simulink model "pr743_QPSK_synch_baseband"  (R2018b)
settings: Solver=VariableStepAuto  StartTime=0.0  StopTime=50000/fs  RelTol=1e-3
PreLoadFcn:
  | Rbit   = 100e3;    % битовая скорость
  | Rsyml = Rbit/2;    % символьная скорость
  | fs = 2.4e6;        % частота дискретизации АЦП
  | interp = fs/Rsyml; % коэффициент передискретизации
  | fc = 600e3;        % несущая частота, Гц
  | fe = 400;          % частотный сдвиг, Гц
  | % параметры контура ФАПЧ
  | T = 1/fs;          % период дискретизации
  | Kp = 1/2;           % КУ ФД
  | Bn = 25000;         % шумовая полоса, Гц
  | Ko = 0.1;          % КУ ГУН
  | d = 0.707;         % демпинг фактор
  | % Коэффициенты ПФ
  | K1 = (4*d*Bn*T)/(Ko*Kp*(d+1/(4*d)));
  | K2 = (4*(Bn*T)^2)/(Ko*Kp*(d+1/4*d)^2);
libraries: commfilt2 x4, commrandsrc3 x1, commdigbbndpm3 x1
settings Model: Creator=Григорий Фокин  LastModifiedBy=Григорий Фокин
settings DataIOCC: SaveFormat=Array  SaveOutput=off  SignalLogging=off  SaveTime=off
settings DebuggingCC: AlgebraicLoopMsg=error
settings HardwareCC: ProdBitPerPointer=32  ProdBitPerSizeT=32  ProdBitPerPtrDiffT=32  ProdLargestAtomicFloat=None  ProdIntDivRoundTo=Undefined  ProdEndianess=Unspecified  ProdWordSize=32  ProdHWDeviceType=ASIC/FPGA->ASIC/FPGA  TargetBitPerPointer=64  TargetBitPerSizeT=64  TargetBitPerPtrDiffT=64  TargetLongLongMode=on  TargetIntDivRoundTo=Zero  TargetEndianess=LittleEndian  TargetWordSize=64  TargetHWDeviceType=Custom Processor->MATLAB Host Computer  ProdEqTarget=off

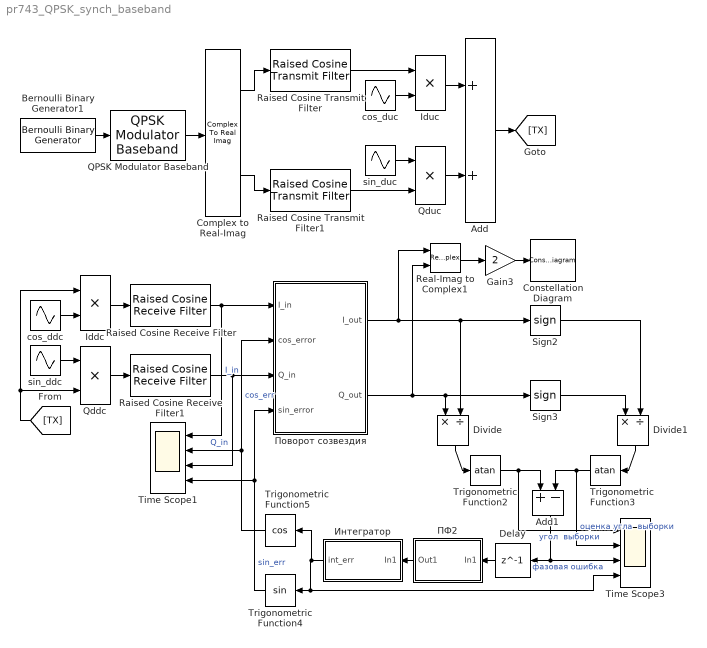
== system pr743_QPSK_synch_baseband ==
  Add : Sum
  Add1 : Sum  Inputs=+-
  Bernoulli Binary Generator1 : commrandsrc3/Bernoulli Binary Generator  ProbabilityOfZero=0.5  SeedSource=Auto  Seed=0  SampleTime=1/Rbit  SamplesPerFrame=2  OutputDataType=double  SimulateUsing=Interpreted execution
  Complex to Real-Imag : ComplexToRealImag
  Constellation Diagram : ConstellationDiagram
  Delay : Delay  DelayLength=1  InitialCondition=0
  Divide : Product  Inputs=*/
  Divide1 : Product  Inputs=*/
  Gain3 : Gain  Gain=2
  Iddc : Product
  Iduc : Product
  QPSK Modulator Baseband : commdigbbndpm3/QPSK Modulator Baseband  InType=Bit  Enc=Gray  Ph=pi/4  outDtype=Fixed-point  outWordLen=16  outUDDataType=sfix(16)  outFracLenMode=Best precision  outFracLen=15  outDataTypeStr=fixdt(1,16)  outLastDataTypeStr=fixdt(1,16)
  Qddc : Product
  Qduc : Product
  Raised Cosine Receive Filter : commfilt2/Raised Cosine Receive Filter  filtType=Square root  R=0.25  filtSpan=8  N=interp  downFactor=interp  downOffset=0  filterGain=1  RateOptions=Allow multirate processing  framing=Mute  checkCoeff=off  variableName=rcRxFilt  currentFiltSpan=8  D=(8)/2  inputOffset=0  sampMode=Mute  saveAsFlag=0  rateMode=Downsampling  checkGain=Normalized  launchFVT=on  roundingMode=Floor  overflowMode=off  coeffDataTypeStr=Inherit: Same word length as input  coeffMin=[]  coeffMax=[]  coeffLastDataTypeStr=Inherit: Same word length as input  accumDataTypeStr=Inherit: Same as product output  accumLastDataTypeStr=Inherit: Same as product output  outputDataTypeStr=Inherit: Same as accumulator  outputMin=[]  outputMax=[]  outputLastDataTypeStr=Inherit: Same as accumulator
  Raised Cosine Receive Filter1 : commfilt2/Raised Cosine Receive Filter  filtType=Square root  R=0.25  filtSpan=8  N=interp  downFactor=interp  downOffset=0  filterGain=1  RateOptions=Allow multirate processing  framing=Mute  checkCoeff=off  variableName=rcRxFilt1  currentFiltSpan=8  D=(8)/2  inputOffset=0  sampMode=Mute  saveAsFlag=0  rateMode=Downsampling  checkGain=Normalized  launchFVT=on  roundingMode=Floor  overflowMode=off  coeffDataTypeStr=Inherit: Same word length as input  coeffMin=[]  coeffMax=[]  coeffLastDataTypeStr=Inherit: Same word length as input  accumDataTypeStr=Inherit: Same as product output  accumLastDataTypeStr=Inherit: Same as product output  outputDataTypeStr=Inherit: Same as accumulator  outputMin=[]  outputMax=[]  outputLastDataTypeStr=Inherit: Same as accumulator
  Raised Cosine Transmit Filter : commfilt2/Raised Cosine Transmit Filter  filtType=Square root  R=0.25  filtSpan=8  N=interp  filterGain=1  RateOptions=Allow multirate processing  framing=Mute  checkCoeff=off  variableName=rcTxFilt  checkGain=Normalized  sampMode=Mute  saveAsFlag=0  currentFiltSpan=8  D=(8)/2  launchFVT=on  roundingMode=Floor  overflowMode=off  coeffDataTypeStr=Inherit: Same word length as input  coeffMin=[]  coeffMax=[]  coeffLastDataTypeStr=Inherit: Same word length as input  outputDataTypeStr=Inherit: Same as accumulator  outputMin=[]  outputMax=[]  outputLastDataTypeStr=Inherit: Same as accumulator
  Raised Cosine Transmit Filter1 : commfilt2/Raised Cosine Transmit Filter  filtType=Square root  R=0.25  filtSpan=8  N=interp  filterGain=1  RateOptions=Allow multirate processing  framing=Mute  checkCoeff=off  variableName=rcTxFilt1  checkGain=Normalized  sampMode=Mute  saveAsFlag=0  currentFiltSpan=8  D=(8)/2  launchFVT=on  roundingMode=Floor  overflowMode=off  coeffDataTypeStr=Inherit: Same word length as input  coeffMin=[]  coeffMax=[]  coeffLastDataTypeStr=Inherit: Same word length as input  outputDataTypeStr=Inherit: Same as accumulator  outputMin=[]  outputMax=[]  outputLastDataTypeStr=Inherit: Same as accumulator
  Real-Imag to Complex1 : RealImagToComplex
  Sign2 : Signum
  Sign3 : Signum
  Time Scope1 : Scope  NumInputPorts=4
  Time Scope3 : Scope  NumInputPorts=4
  Trigonometric Function2 : Trigonometry  Operator=atan  OutputSignalType=real
  Trigonometric Function3 : Trigonometry  Operator=atan  OutputSignalType=real
  Trigonometric Function4 : Trigonometry
  Trigonometric Function5 : Trigonometry  Operator=cos
  cos_ddc : Sin  Frequency=fc*2*pi  Phase=pi/2  SampleTime=1/fs
  cos_duc : Sin  Frequency=(fc+fe)*2*pi  Phase=pi/2  SampleTime=1/fs
  sin_ddc : Sin  Frequency=fc*2*pi  SampleTime=1/fs
  sin_duc : Sin  Frequency=(fc+fe)*2*pi  SampleTime=1/fs
  Интегратор : Subsystem
  ПФ2 : Subsystem
  "Поворот созвездия " : Subsystem
  wires:
  cos_duc/1 -> Iduc/2
  Complex to Real-Imag/1 -> Raised Cosine Transmit Filter/1
  Qduc/1 -> Add/2
  Iduc/1 -> Add/1
  QPSK Modulator Baseband/1 -> Complex to Real-Imag/1
  Bernoulli Binary Generator1/1 -> QPSK Modulator Baseband/1
  sin_duc/1 -> Qduc/1
  Raised Cosine Transmit Filter/1 -> Iduc/1
  Raised Cosine Transmit Filter1/1 -> Qduc/2
  Add/1 -> [TX]
  [TX] -> Iddc/1, Qddc/2
  sin_ddc/1 -> Qddc/1
  cos_ddc/1 -> Iddc/2
  Iddc/1 -> Raised Cosine Receive Filter/1
  Qddc/1 -> Raised Cosine Receive Filter1/1
  Complex to Real-Imag/2 -> Raised Cosine Transmit Filter1/1
  Raised Cosine Receive Filter/1 -> Time Scope1/1, "Поворот созвездия "/1(I_in)  "I_in"
  Raised Cosine Receive Filter1/1 -> "Поворот созвездия "/3(Q_in), Time Scope1/3  "Q_in"
  ПФ2/1(Out1) -> Интегратор/1(In1)
  Delay/1 -> ПФ2/1(In1)
  "Поворот созвездия "/1(I_out) -> Real-Imag to Complex1/1, Divide/2, Sign2/1
  "Поворот созвездия "/2(Q_out) -> Divide/1, Sign3/1, Real-Imag to Complex1/2
  Sign2/1 -> Divide1/2
  Sign3/1 -> Divide1/1
  Divide/1 -> Trigonometric Function2/1
  Divide1/1 -> Trigonometric Function3/1
  Trigonometric Function2/1 -> Add1/1, Time Scope3/1  "угол  выборки"
  Trigonometric Function3/1 -> Add1/2, Time Scope3/2  "оценка угла  выборки"
  Add1/1 -> Time Scope3/3, Delay/1  "фазовая ошибка"
  Gain3/1 -> Constellation Diagram/1
  Real-Imag to Complex1/1 -> Gain3/1
  Интегратор/1(int_err) -> Trigonometric Function5/1, Trigonometric Function4/1, Time Scope3/4
  Trigonometric Function5/1 -> Time Scope1/2, "Поворот созвездия "/2(cos_error)  "cos_err"
  Trigonometric Function4/1 -> Time Scope1/4, "Поворот созвездия "/4(sin_error)  "sin_err"

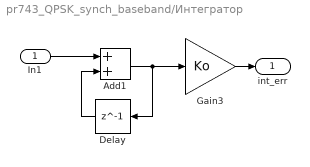
== system pr743_QPSK_synch_baseband/Интегратор ==
  In1 : Inport
  Add1 : Sum
  Delay : Delay  DelayLength=1
  Gain3 : Gain  Gain=Ko
  int_err : Outport
  wires:
  Add1/1 -> Delay/1, Gain3/1
  Delay/1 -> Add1/2
  In1/1 -> Add1/1
  Gain3/1 -> int_err/1

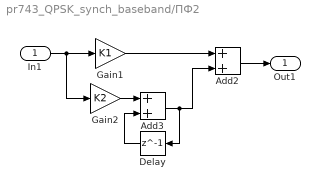
== system pr743_QPSK_synch_baseband/ПФ2 ==
  In1 : Inport
  Add2 : Sum
  Add3 : Sum
  Delay : Delay  DelayLength=1  InitialCondition=0
  Gain1 : Gain  Gain=K1
  Gain2 : Gain  Gain=K2
  Out1 : Outport
  wires:
  Delay/1 -> Add3/2
  Add2/1 -> Out1/1
  Gain2/1 -> Add3/1
  In1/1 -> Gain2/1, Gain1/1
  Add3/1 -> Delay/1, Add2/2
  Gain1/1 -> Add2/1

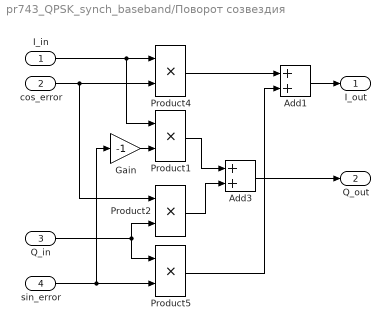
== system pr743_QPSK_synch_baseband/Поворот созвездия  ==
  I_in : Inport
  cos_error : Inport  Port=2
  Q_in : Inport  Port=3
  sin_error : Inport  Port=4
  Add1 : Sum
  Add3 : Sum
  Gain : Gain  Gain=-1
  Product{1..2,4..5} (4 alike) : Product
  I_out : Outport
  Q_out : Outport  Port=2
  wires:
  I_in/1 -> Product1/1, Product4/1
  cos_error/1 -> Product2/1, Product4/2
  sin_error/1 -> Gain/1, Product5/2
  Product5/1 -> Add1/2
  Product4/1 -> Add1/1
  Product2/1 -> Add3/2
  Gain/1 -> Product1/2
  Add1/1 -> I_out/1
  Q_in/1 -> Product5/1, Product2/2
  Product1/1 -> Add3/1
  Add3/1 -> Q_out/1
